simulink model "find_y"  (R2022b)
settings: Solver=VariableStepAuto  StartTime=0.0  StopTime=25  MaxStep=0.01  RelTol=1e-3
settings Model: Creator=Brigosha_Guest  LastModifiedBy=Brigosha_Guest

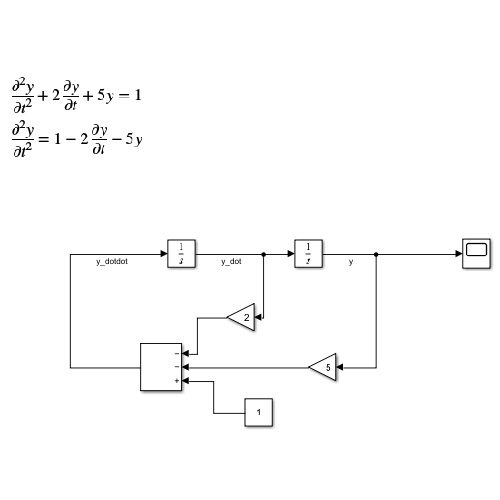
[thumbnail: Simulink's stored preview of the top-level diagram]
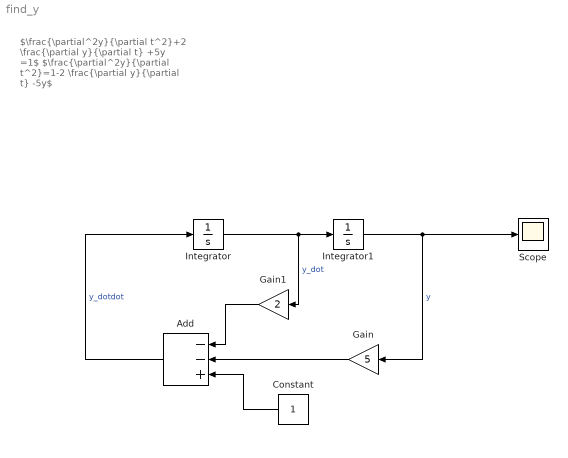
== system find_y ==
  note: $\frac{\partial^2y}{\partial t^2}+2 \frac{\partial y}{\partial t} +5y =1$
      | $\frac{\partial^2y}{\partial t^2}=1-2 \frac{\partial y}{\partial t} -5y$
  Add : Sum  Inputs=--+
  Constant : Constant
  Gain : Gain  Gain=5
  Gain1 : Gain  Gain=2
  Integrator : Integrator
  Integrator1 : Integrator
  Scope : Scope
  wires:
  Add/1 -> Integrator/1  "y_dotdot"
  Integrator/1 -> Gain1/1, Integrator1/1  "y_dot"
  Integrator1/1 -> Gain/1, Scope/1  "y"
  Gain1/1 -> Add/1
  Gain/1 -> Add/2
  Constant/1 -> Add/3
